simulink model "CORDIC"  (R2021a)
settings: Solver=VariableStepAuto  StartTime=0.0  StopTime=400  RelTol=1e-3
undefined symbols (not defined in the file or in its folder): AXI4, Lite
libraries: hdlBasic x776, xbsIndex_r4 x1
(part 7 of 7)

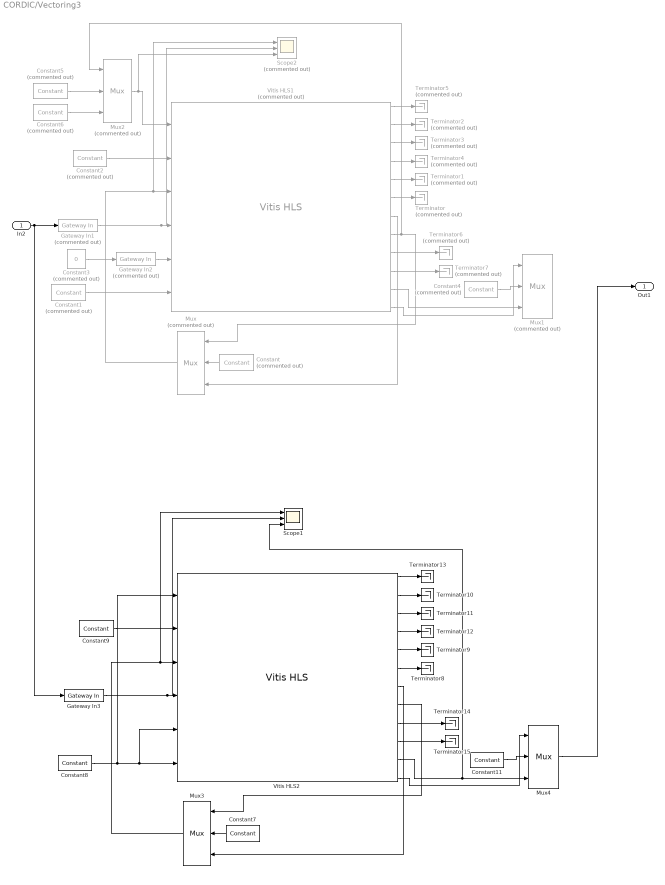
== system CORDIC/Vectoring3 ==
  In2 : Inport
  Constant : hdlBasic/Constant  Commented=on  const=0  gui_display_data_type=Fixed-point  arith_type=Signed (2's comp)  n_bits=16  bin_pt=13  preci_type=Single  exp_width=8  frac_width=24  explicit_period=off  period=1  XmcBlockStatus=1  maskContainerNames=tabcontainer1  block_type=constant  block_config=sysgen:Constant_config
  Constant1 : hdlBasic/Constant  Commented=on  const=0  gui_display_data_type=Boolean  arith_type=Boolean  n_bits=16  bin_pt=13  preci_type=Single  exp_width=8  frac_width=24  explicit_period=off  period=1  XmcBlockStatus=1  maskContainerNames=tabcontainer1  block_type=constant  block_config=sysgen:Constant_config
  Constant11 : hdlBasic/Constant  const=0  gui_display_data_type=Fixed-point  arith_type=Signed (2's comp)  n_bits=16  bin_pt=13  preci_type=Single  exp_width=8  frac_width=24  explicit_period=off  period=1  XmcBlockStatus=1  maskContainerNames=tabcontainer1  block_type=constant  block_config=sysgen:Constant_config
  Constant2 : hdlBasic/Constant  Commented=on  const=1  gui_display_data_type=Boolean  arith_type=Boolean  n_bits=16  bin_pt=13  preci_type=Single  exp_width=8  frac_width=24  explicit_period=off  period=1  XmcBlockStatus=1  maskContainerNames=tabcontainer1  block_type=constant  block_config=sysgen:Constant_config
  Constant3 : Constant  Commented=on  Value=0
  Constant4 : hdlBasic/Constant  Commented=on  const=0  gui_display_data_type=Fixed-point  arith_type=Signed (2's comp)  n_bits=16  bin_pt=13  preci_type=Single  exp_width=8  frac_width=24  explicit_period=off  period=1  XmcBlockStatus=1  maskContainerNames=tabcontainer1  block_type=constant  block_config=sysgen:Constant_config
  Constant5 : hdlBasic/Constant  Commented=on  const=0  gui_display_data_type=Boolean  arith_type=Boolean  n_bits=16  bin_pt=14  preci_type=Single  exp_width=8  frac_width=24  explicit_period=off  period=1  XmcBlockStatus=1  maskContainerNames=tabcontainer1  block_type=constant  block_config=sysgen:Constant_config
  Constant6 : hdlBasic/Constant  Commented=on  const=1.0  gui_display_data_type=Boolean  arith_type=Boolean  n_bits=16  bin_pt=14  preci_type=Single  exp_width=8  frac_width=24  explicit_period=off  period=1  XmcBlockStatus=1  maskContainerNames=tabcontainer1  block_type=constant  block_config=sysgen:Constant_config
  Constant7 : hdlBasic/Constant  const=0  gui_display_data_type=Fixed-point  arith_type=Signed (2's comp)  n_bits=16  bin_pt=13  preci_type=Single  exp_width=8  frac_width=24  explicit_period=off  period=1  XmcBlockStatus=1  maskContainerNames=tabcontainer1  block_type=constant  block_config=sysgen:Constant_config
  Constant8 : hdlBasic/Constant  const=0  gui_display_data_type=Boolean  arith_type=Boolean  n_bits=16  bin_pt=13  preci_type=Single  exp_width=8  frac_width=24  explicit_period=off  period=1  XmcBlockStatus=1  maskContainerNames=tabcontainer1  block_type=constant  block_config=sysgen:Constant_config
  Constant9 : hdlBasic/Constant  const=1  gui_display_data_type=Boolean  arith_type=Boolean  n_bits=16  bin_pt=13  preci_type=Single  exp_width=8  frac_width=24  explicit_period=off  period=1  XmcBlockStatus=1  maskContainerNames=tabcontainer1  block_type=constant  block_config=sysgen:Constant_config
  Gateway In1 : hdlBasic/Gateway In  Commented=on  gui_display_data_type=Fixed-point  arith_type=Signed (2's comp)  n_bits=16  bin_pt=13  preci_type=Single  exp_width=8  frac_width=24  rows=1  columns=1  quantization="Round  (unbiased: +/- Inf)"  overflow=Saturate  period=1  UseAsADC=off  ADCChannel='1'  interface=None  automatic_assignment=on  address_offset=hex2dec('00')  intf_name=''  intf_description=''  default_value=0  timing_constraint=None  locs_specified=off  LOCs={}  io_standard={}  inherit_from_input=off  hdl_port=on  XmcBlockStatus=1  maskContainerNames=group4  block_type=gatewayin  block_config=sysgen:gateway_in_config  block_width_w=590  block_height_w=620  block_width=640  block_height=850
  Gateway In2 : hdlBasic/Gateway In  Commented=on  gui_display_data_type=Fixed-point  arith_type=Signed (2's comp)  n_bits=16  bin_pt=13  preci_type=Single  exp_width=8  frac_width=24  rows=1  columns=1  quantization="Round  (unbiased: +/- Inf)"  overflow=Saturate  period=1  UseAsADC=off  ADCChannel='1'  interface=None  automatic_assignment=on  address_offset=hex2dec('00')  intf_name=''  intf_description=''  default_value=0  timing_constraint=None  locs_specified=off  LOCs={}  io_standard={}  inherit_from_input=off  hdl_port=on  XmcBlockStatus=1  maskContainerNames=group4  block_type=gatewayin  block_config=sysgen:gateway_in_config  block_width_w=590  block_height_w=620  block_width=640  block_height=850
  Gateway In3 : hdlBasic/Gateway In  gui_display_data_type=Fixed-point  arith_type=Signed (2's comp)  n_bits=16  bin_pt=13  preci_type=Single  exp_width=8  frac_width=24  rows=1  columns=1  quantization="Round  (unbiased: +/- Inf)"  overflow=Saturate  period=1  UseAsADC=off  ADCChannel='1'  interface=None  automatic_assignment=on  address_offset=hex2dec('00')  intf_name=''  intf_description=''  default_value=0  timing_constraint=None  locs_specified=off  LOCs={}  io_standard={}  inherit_from_input=off  hdl_port=on  XmcBlockStatus=1  maskContainerNames=group4  block_type=gatewayin  block_config=sysgen:gateway_in_config  block_width_w=590  block_height_w=620  block_width=640  block_height=850
  Mux : hdlBasic/Mux  Commented=on  inputs=2  en=off  latency=1  precision=Full  arith_type=Unsigned  n_bits=16  bin_pt=14  quantization=Truncate  overflow=Wrap  XmcBlockStatus=1  maskContainerNames=tabcontainer1  block_type=mux  block_config=sysgen:Mux_config
  Mux1 : hdlBasic/Mux  Commented=on  inputs=2  en=off  latency=1  precision=Full  arith_type=Unsigned  n_bits=16  bin_pt=14  quantization=Truncate  overflow=Wrap  XmcBlockStatus=1  maskContainerNames=tabcontainer1  block_type=mux  block_config=sysgen:Mux_config
  Mux2 : hdlBasic/Mux  Commented=on  inputs=2  en=off  latency=1  precision=Full  arith_type=Unsigned  n_bits=16  bin_pt=14  quantization=Truncate  overflow=Wrap  XmcBlockStatus=1  maskContainerNames=tabcontainer1  block_type=mux  block_config=sysgen:Mux_config
  Mux3 : hdlBasic/Mux  inputs=2  en=off  latency=1  precision=Full  arith_type=Unsigned  n_bits=16  bin_pt=14  quantization=Truncate  overflow=Wrap  XmcBlockStatus=1  maskContainerNames=tabcontainer1  block_type=mux  block_config=sysgen:Mux_config
  Mux4 : hdlBasic/Mux  inputs=2  en=off  latency=1  precision=Full  arith_type=Unsigned  n_bits=16  bin_pt=14  quantization=Truncate  overflow=Wrap  XmcBlockStatus=1  maskContainerNames=tabcontainer1  block_type=mux  block_config=sysgen:Mux_config
  Scope1 : Scope  NumInputPorts=3
  Scope2 : Scope  Commented=on  NumInputPorts=3
  Terminator{,1..7} (8 alike) : Terminator  Commented=on
  Terminator{8..15} (8 alike) : Terminator
  Vitis HLS1 : hdlBasic/Vitis HLS  Commented=on  anytable='C:\ELEC522\jz118\HLS\cordic\solution1'  fast_sim=off  display_datatype=off  rate_propagation_method=Simulink system period  model_file_path=''  latency=1  block_type=vitis_hls
      settings: infoedit=This block allows including C,C++ and SystemC source files in System Generator for DSP designs.
  Vitis HLS2 : hdlBasic/Vitis HLS  anytable='C:\ELEC522\jz118\HLS\cordic\solution1'  fast_sim=off  display_datatype=off  rate_propagation_method=Simulink system period  model_file_path=''  latency=1  block_type=vitis_hls
      settings: infoedit=This block allows including C,C++ and SystemC source files in System Generator for DSP designs.
  Out1 : Outport
  wires:
  Gateway In2/1 -> Vitis HLS1/5
  In2/1 -> Gateway In1/1, Gateway In3/1
  Gateway In1/1 -> Scope2/2, Vitis HLS1/4
  Constant3/1 -> Gateway In2/1
  Constant2/1 -> Vitis HLS1/2
  Vitis HLS1/8 -> Mux/1, Mux2/1
  Mux/1 -> Scope2/1, Vitis HLS1/3
  Constant/1 -> Mux/2
  Vitis HLS1/7 -> Mux/3
  Vitis HLS1/6 -> Terminator/1
  Vitis HLS1/5 -> Terminator1/1
  Vitis HLS1/2 -> Terminator2/1
  Vitis HLS1/3 -> Terminator3/1
  Vitis HLS1/4 -> Terminator4/1
  Vitis HLS1/1 -> Terminator5/1
  Vitis HLS1/9 -> Terminator6/1
  Vitis HLS1/10 -> Terminator7/1
  Vitis HLS1/11 -> Mux1/3
  Constant4/1 -> Mux1/2
  Vitis HLS1/12 -> Mux1/1
  Constant6/1 -> Mux2/3
  Constant5/1 -> Mux2/2
  Constant1/1 -> Vitis HLS1/6
  Mux2/1 -> Scope2/3, Vitis HLS1/1
  Constant11/1 -> Mux4/2
  Vitis HLS2/11 -> Scope1/3, Mux4/3
  Vitis HLS2/12 -> Mux4/1
  Vitis HLS2/9 -> Terminator14/1
  Vitis HLS2/5 -> Terminator9/1
  Vitis HLS2/2 -> Terminator10/1
  Vitis HLS2/4 -> Terminator12/1
  Vitis HLS2/6 -> Terminator8/1
  Vitis HLS2/10 -> Terminator15/1
  Constant7/1 -> Mux3/2
  Constant8/1 -> Vitis HLS2/1, Vitis HLS2/5, Vitis HLS2/6
  Mux3/1 -> Scope1/1, Vitis HLS2/3
  Vitis HLS2/7 -> Mux3/3
  Vitis HLS2/8 -> Mux3/1
  Gateway In3/1 -> Scope1/2, Vitis HLS2/4
  Constant9/1 -> Vitis HLS2/2
  Vitis HLS2/3 -> Terminator11/1
  Vitis HLS2/1 -> Terminator13/1
  Mux4/1 -> Out1/1

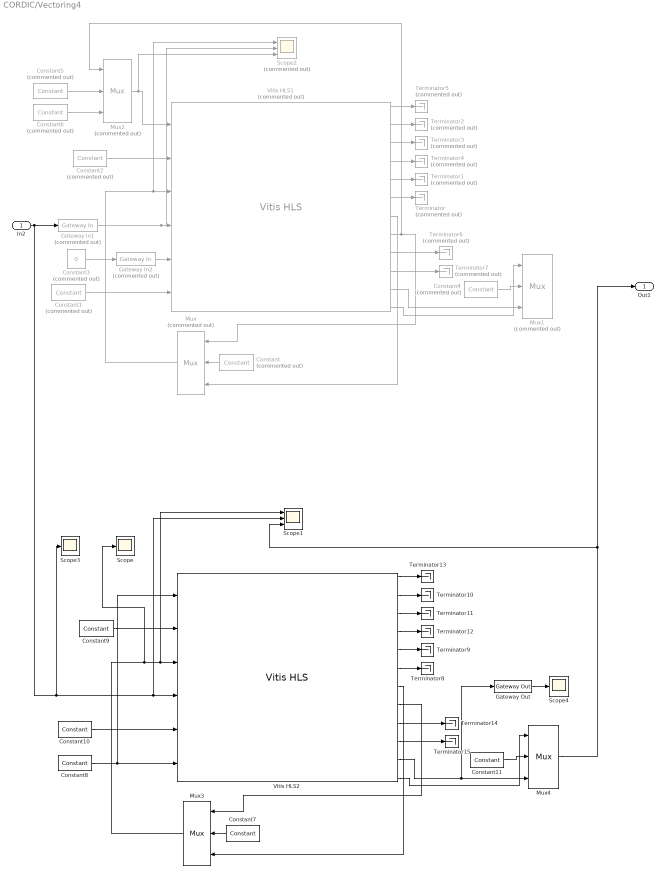
== system CORDIC/Vectoring4 ==
  In2 : Inport
  Constant : hdlBasic/Constant  Commented=on  const=0  gui_display_data_type=Fixed-point  arith_type=Signed (2's comp)  n_bits=16  bin_pt=13  preci_type=Single  exp_width=8  frac_width=24  explicit_period=off  period=1  XmcBlockStatus=1  maskContainerNames=tabcontainer1  block_type=constant  block_config=sysgen:Constant_config
  Constant1 : hdlBasic/Constant  Commented=on  const=0  gui_display_data_type=Boolean  arith_type=Boolean  n_bits=16  bin_pt=13  preci_type=Single  exp_width=8  frac_width=24  explicit_period=off  period=1  XmcBlockStatus=1  maskContainerNames=tabcontainer1  block_type=constant  block_config=sysgen:Constant_config
  Constant10 : hdlBasic/Constant  const=0  gui_display_data_type=Fixed-point  arith_type=Signed (2's comp)  n_bits=16  bin_pt=13  preci_type=Single  exp_width=8  frac_width=24  explicit_period=off  period=1  XmcBlockStatus=1  maskContainerNames=tabcontainer1  block_type=constant  block_config=sysgen:Constant_config
  Constant11 : hdlBasic/Constant  const=0  gui_display_data_type=Fixed-point  arith_type=Signed (2's comp)  n_bits=16  bin_pt=13  preci_type=Single  exp_width=8  frac_width=24  explicit_period=off  period=1  XmcBlockStatus=1  maskContainerNames=tabcontainer1  block_type=constant  block_config=sysgen:Constant_config
  Constant2 : hdlBasic/Constant  Commented=on  const=1  gui_display_data_type=Boolean  arith_type=Boolean  n_bits=16  bin_pt=13  preci_type=Single  exp_width=8  frac_width=24  explicit_period=off  period=1  XmcBlockStatus=1  maskContainerNames=tabcontainer1  block_type=constant  block_config=sysgen:Constant_config
  Constant3 : Constant  Commented=on  Value=0
  Constant4 : hdlBasic/Constant  Commented=on  const=0  gui_display_data_type=Fixed-point  arith_type=Signed (2's comp)  n_bits=16  bin_pt=13  preci_type=Single  exp_width=8  frac_width=24  explicit_period=off  period=1  XmcBlockStatus=1  maskContainerNames=tabcontainer1  block_type=constant  block_config=sysgen:Constant_config
  Constant5 : hdlBasic/Constant  Commented=on  const=0  gui_display_data_type=Boolean  arith_type=Boolean  n_bits=16  bin_pt=14  preci_type=Single  exp_width=8  frac_width=24  explicit_period=off  period=1  XmcBlockStatus=1  maskContainerNames=tabcontainer1  block_type=constant  block_config=sysgen:Constant_config
  Constant6 : hdlBasic/Constant  Commented=on  const=1.0  gui_display_data_type=Boolean  arith_type=Boolean  n_bits=16  bin_pt=14  preci_type=Single  exp_width=8  frac_width=24  explicit_period=off  period=1  XmcBlockStatus=1  maskContainerNames=tabcontainer1  block_type=constant  block_config=sysgen:Constant_config
  Constant7 : hdlBasic/Constant  const=0  gui_display_data_type=Fixed-point  arith_type=Signed (2's comp)  n_bits=16  bin_pt=13  preci_type=Single  exp_width=8  frac_width=24  explicit_period=off  period=1  XmcBlockStatus=1  maskContainerNames=tabcontainer1  block_type=constant  block_config=sysgen:Constant_config
  Constant8 : hdlBasic/Constant  const=0  gui_display_data_type=Boolean  arith_type=Boolean  n_bits=16  bin_pt=13  preci_type=Single  exp_width=8  frac_width=24  explicit_period=off  period=1  XmcBlockStatus=1  maskContainerNames=tabcontainer1  block_type=constant  block_config=sysgen:Constant_config
  Constant9 : hdlBasic/Constant  const=1  gui_display_data_type=Boolean  arith_type=Boolean  n_bits=16  bin_pt=13  preci_type=Single  exp_width=8  frac_width=24  explicit_period=off  period=1  XmcBlockStatus=1  maskContainerNames=tabcontainer1  block_type=constant  block_config=sysgen:Constant_config
  Gateway In1 : hdlBasic/Gateway In  Commented=on  gui_display_data_type=Fixed-point  arith_type=Signed (2's comp)  n_bits=16  bin_pt=13  preci_type=Single  exp_width=8  frac_width=24  rows=1  columns=1  quantization="Round  (unbiased: +/- Inf)"  overflow=Saturate  period=1  UseAsADC=off  ADCChannel='1'  interface=None  automatic_assignment=on  address_offset=hex2dec('00')  intf_name=''  intf_description=''  default_value=0  timing_constraint=None  locs_specified=off  LOCs={}  io_standard={}  inherit_from_input=off  hdl_port=on  XmcBlockStatus=1  maskContainerNames=group4  block_type=gatewayin  block_config=sysgen:gateway_in_config  block_width_w=590  block_height_w=620  block_width=640  block_height=850
  Gateway In2 : hdlBasic/Gateway In  Commented=on  gui_display_data_type=Fixed-point  arith_type=Signed (2's comp)  n_bits=16  bin_pt=13  preci_type=Single  exp_width=8  frac_width=24  rows=1  columns=1  quantization="Round  (unbiased: +/- Inf)"  overflow=Saturate  period=1  UseAsADC=off  ADCChannel='1'  interface=None  automatic_assignment=on  address_offset=hex2dec('00')  intf_name=''  intf_description=''  default_value=0  timing_constraint=None  locs_specified=off  LOCs={}  io_standard={}  inherit_from_input=off  hdl_port=on  XmcBlockStatus=1  maskContainerNames=group4  block_type=gatewayin  block_config=sysgen:gateway_in_config  block_width_w=590  block_height_w=620  block_width=640  block_height=850
  Gateway Out : hdlBasic/Gateway Out  inherit_from_input=off  hdl_port=on  rows=1  columns=1  UseAsDAC=off  DACChannel='1'  interface=None  automatic_assignment=on  address_offset=hex2dec('00')  intf_name=''  intf_description=''  timing_constraint=None  locs_specified=off  LOCs={}  io_standard={}  XmcBlockStatus=1  maskContainerNames=group4  block_type=gatewayout  block_config=sysgen:gateway_out_config  block_width_w=590  block_height_w=620  block_width=620  block_height=750
  Mux : hdlBasic/Mux  Commented=on  inputs=2  en=off  latency=1  precision=Full  arith_type=Unsigned  n_bits=16  bin_pt=14  quantization=Truncate  overflow=Wrap  XmcBlockStatus=1  maskContainerNames=tabcontainer1  block_type=mux  block_config=sysgen:Mux_config
  Mux1 : hdlBasic/Mux  Commented=on  inputs=2  en=off  latency=1  precision=Full  arith_type=Unsigned  n_bits=16  bin_pt=14  quantization=Truncate  overflow=Wrap  XmcBlockStatus=1  maskContainerNames=tabcontainer1  block_type=mux  block_config=sysgen:Mux_config
  Mux2 : hdlBasic/Mux  Commented=on  inputs=2  en=off  latency=1  precision=Full  arith_type=Unsigned  n_bits=16  bin_pt=14  quantization=Truncate  overflow=Wrap  XmcBlockStatus=1  maskContainerNames=tabcontainer1  block_type=mux  block_config=sysgen:Mux_config
  Mux3 : hdlBasic/Mux  inputs=2  en=off  latency=1  precision=Full  arith_type=Unsigned  n_bits=16  bin_pt=14  quantization=Truncate  overflow=Wrap  XmcBlockStatus=1  maskContainerNames=tabcontainer1  block_type=mux  block_config=sysgen:Mux_config
  Mux4 : hdlBasic/Mux  inputs=2  en=off  latency=1  precision=Full  arith_type=Unsigned  n_bits=16  bin_pt=14  quantization=Truncate  overflow=Wrap  XmcBlockStatus=1  maskContainerNames=tabcontainer1  block_type=mux  block_config=sysgen:Mux_config
  Scope : Scope
  Scope1 : Scope  NumInputPorts=3
  Scope2 : Scope  Commented=on  NumInputPorts=3
  Scope3 : Scope
  Scope4 : Scope
  Terminator{,1..7} (8 alike) : Terminator  Commented=on
  Terminator{8..15} (8 alike) : Terminator
  Vitis HLS1 : hdlBasic/Vitis HLS  Commented=on  anytable='C:\ELEC522\jz118\HLS\cordic\solution1'  fast_sim=off  display_datatype=off  rate_propagation_method=Simulink system period  model_file_path=''  latency=1  block_type=vitis_hls
      settings: infoedit=This block allows including C,C++ and SystemC source files in System Generator for DSP designs.
  Vitis HLS2 : hdlBasic/Vitis HLS  anytable='C:\ELEC522\jz118\HLS\cordic\solution1'  fast_sim=off  display_datatype=off  rate_propagation_method=Simulink system period  model_file_path=''  latency=1  block_type=vitis_hls
      settings: infoedit=This block allows including C,C++ and SystemC source files in System Generator for DSP designs.
  Out1 : Outport
  wires:
  Gateway In2/1 -> Vitis HLS1/5
  Gateway In1/1 -> Scope2/2, Vitis HLS1/4
  Constant3/1 -> Gateway In2/1
  Constant2/1 -> Vitis HLS1/2
  Vitis HLS1/8 -> Mux/1, Mux2/1
  Mux/1 -> Scope2/1, Vitis HLS1/3
  Constant/1 -> Mux/2
  Vitis HLS1/7 -> Mux/3
  Vitis HLS1/6 -> Terminator/1
  Vitis HLS1/5 -> Terminator1/1
  Vitis HLS1/2 -> Terminator2/1
  Vitis HLS1/3 -> Terminator3/1
  Vitis HLS1/4 -> Terminator4/1
  Vitis HLS1/1 -> Terminator5/1
  Vitis HLS1/9 -> Terminator6/1
  Vitis HLS1/10 -> Terminator7/1
  Vitis HLS1/11 -> Mux1/3
  Constant4/1 -> Mux1/2
  Vitis HLS1/12 -> Mux1/1
  Constant6/1 -> Mux2/3
  Constant5/1 -> Mux2/2
  Constant1/1 -> Vitis HLS1/6
  Mux2/1 -> Scope2/3, Vitis HLS1/1
  Constant11/1 -> Mux4/2
  Vitis HLS2/11 -> Gateway Out/1, Mux4/3
  Vitis HLS2/12 -> Mux4/1
  Vitis HLS2/9 -> Terminator14/1
  Vitis HLS2/5 -> Terminator9/1
  Vitis HLS2/2 -> Terminator10/1
  Vitis HLS2/4 -> Terminator12/1
  Vitis HLS2/6 -> Terminator8/1
  Vitis HLS2/10 -> Terminator15/1
  Constant7/1 -> Mux3/2
  Constant8/1 -> Vitis HLS2/1, Vitis HLS2/6
  Mux3/1 -> Scope/1, Scope1/1, Vitis HLS2/3
  Vitis HLS2/7 -> Mux3/3
  Vitis HLS2/8 -> Mux3/1
  Constant9/1 -> Vitis HLS2/2
  Vitis HLS2/3 -> Terminator11/1
  Vitis HLS2/1 -> Terminator13/1
  Mux4/1 -> Scope1/3, Out1/1
  Constant10/1 -> Vitis HLS2/5
  Gateway Out/1 -> Scope4/1
  In2/1 -> Scope1/2, Vitis HLS2/4, Scope3/1, Gateway In1/1

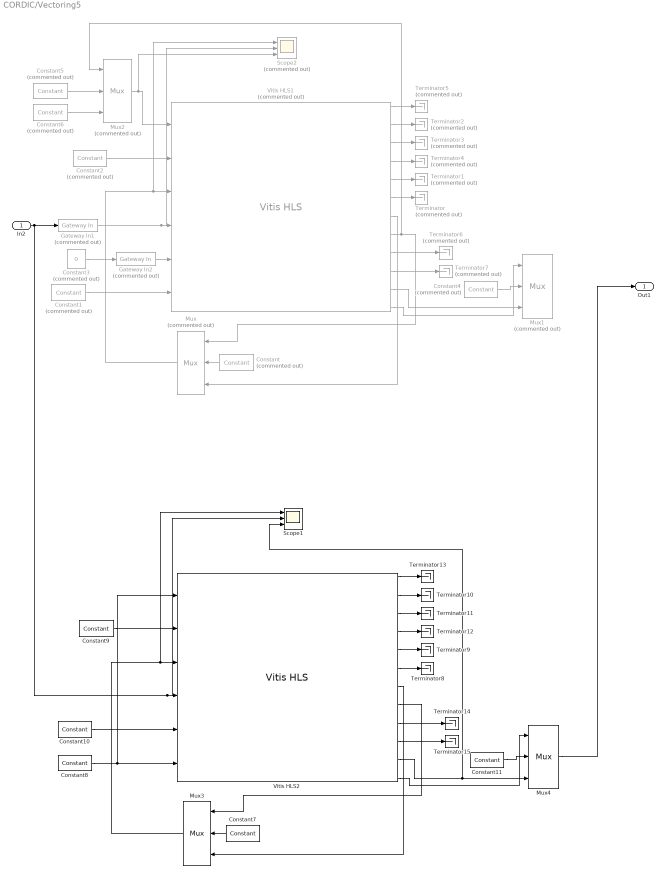
== system CORDIC/Vectoring5 ==
  In2 : Inport
  Constant : hdlBasic/Constant  Commented=on  const=0  gui_display_data_type=Fixed-point  arith_type=Signed (2's comp)  n_bits=16  bin_pt=13  preci_type=Single  exp_width=8  frac_width=24  explicit_period=off  period=1  XmcBlockStatus=1  maskContainerNames=tabcontainer1  block_type=constant  block_config=sysgen:Constant_config
  Constant1 : hdlBasic/Constant  Commented=on  const=0  gui_display_data_type=Boolean  arith_type=Boolean  n_bits=16  bin_pt=13  preci_type=Single  exp_width=8  frac_width=24  explicit_period=off  period=1  XmcBlockStatus=1  maskContainerNames=tabcontainer1  block_type=constant  block_config=sysgen:Constant_config
  Constant10 : hdlBasic/Constant  const=0  gui_display_data_type=Fixed-point  arith_type=Signed (2's comp)  n_bits=16  bin_pt=13  preci_type=Single  exp_width=8  frac_width=24  explicit_period=off  period=1  XmcBlockStatus=1  maskContainerNames=tabcontainer1  block_type=constant  block_config=sysgen:Constant_config
  Constant11 : hdlBasic/Constant  const=0  gui_display_data_type=Fixed-point  arith_type=Signed (2's comp)  n_bits=16  bin_pt=13  preci_type=Single  exp_width=8  frac_width=24  explicit_period=off  period=1  XmcBlockStatus=1  maskContainerNames=tabcontainer1  block_type=constant  block_config=sysgen:Constant_config
  Constant2 : hdlBasic/Constant  Commented=on  const=1  gui_display_data_type=Boolean  arith_type=Boolean  n_bits=16  bin_pt=13  preci_type=Single  exp_width=8  frac_width=24  explicit_period=off  period=1  XmcBlockStatus=1  maskContainerNames=tabcontainer1  block_type=constant  block_config=sysgen:Constant_config
  Constant3 : Constant  Commented=on  Value=0
  Constant4 : hdlBasic/Constant  Commented=on  const=0  gui_display_data_type=Fixed-point  arith_type=Signed (2's comp)  n_bits=16  bin_pt=13  preci_type=Single  exp_width=8  frac_width=24  explicit_period=off  period=1  XmcBlockStatus=1  maskContainerNames=tabcontainer1  block_type=constant  block_config=sysgen:Constant_config
  Constant5 : hdlBasic/Constant  Commented=on  const=0  gui_display_data_type=Boolean  arith_type=Boolean  n_bits=16  bin_pt=14  preci_type=Single  exp_width=8  frac_width=24  explicit_period=off  period=1  XmcBlockStatus=1  maskContainerNames=tabcontainer1  block_type=constant  block_config=sysgen:Constant_config
  Constant6 : hdlBasic/Constant  Commented=on  const=1.0  gui_display_data_type=Boolean  arith_type=Boolean  n_bits=16  bin_pt=14  preci_type=Single  exp_width=8  frac_width=24  explicit_period=off  period=1  XmcBlockStatus=1  maskContainerNames=tabcontainer1  block_type=constant  block_config=sysgen:Constant_config
  Constant7 : hdlBasic/Constant  const=0  gui_display_data_type=Fixed-point  arith_type=Signed (2's comp)  n_bits=16  bin_pt=13  preci_type=Single  exp_width=8  frac_width=24  explicit_period=off  period=1  XmcBlockStatus=1  maskContainerNames=tabcontainer1  block_type=constant  block_config=sysgen:Constant_config
  Constant8 : hdlBasic/Constant  const=0  gui_display_data_type=Boolean  arith_type=Boolean  n_bits=16  bin_pt=13  preci_type=Single  exp_width=8  frac_width=24  explicit_period=off  period=1  XmcBlockStatus=1  maskContainerNames=tabcontainer1  block_type=constant  block_config=sysgen:Constant_config
  Constant9 : hdlBasic/Constant  const=1  gui_display_data_type=Boolean  arith_type=Boolean  n_bits=16  bin_pt=13  preci_type=Single  exp_width=8  frac_width=24  explicit_period=off  period=1  XmcBlockStatus=1  maskContainerNames=tabcontainer1  block_type=constant  block_config=sysgen:Constant_config
  Gateway In1 : hdlBasic/Gateway In  Commented=on  gui_display_data_type=Fixed-point  arith_type=Signed (2's comp)  n_bits=16  bin_pt=13  preci_type=Single  exp_width=8  frac_width=24  rows=1  columns=1  quantization="Round  (unbiased: +/- Inf)"  overflow=Saturate  period=1  UseAsADC=off  ADCChannel='1'  interface=None  automatic_assignment=on  address_offset=hex2dec('00')  intf_name=''  intf_description=''  default_value=0  timing_constraint=None  locs_specified=off  LOCs={}  io_standard={}  inherit_from_input=off  hdl_port=on  XmcBlockStatus=1  maskContainerNames=group4  block_type=gatewayin  block_config=sysgen:gateway_in_config  block_width_w=590  block_height_w=620  block_width=640  block_height=850
  Gateway In2 : hdlBasic/Gateway In  Commented=on  gui_display_data_type=Fixed-point  arith_type=Signed (2's comp)  n_bits=16  bin_pt=13  preci_type=Single  exp_width=8  frac_width=24  rows=1  columns=1  quantization="Round  (unbiased: +/- Inf)"  overflow=Saturate  period=1  UseAsADC=off  ADCChannel='1'  interface=None  automatic_assignment=on  address_offset=hex2dec('00')  intf_name=''  intf_description=''  default_value=0  timing_constraint=None  locs_specified=off  LOCs={}  io_standard={}  inherit_from_input=off  hdl_port=on  XmcBlockStatus=1  maskContainerNames=group4  block_type=gatewayin  block_config=sysgen:gateway_in_config  block_width_w=590  block_height_w=620  block_width=640  block_height=850
  Mux : hdlBasic/Mux  Commented=on  inputs=2  en=off  latency=1  precision=Full  arith_type=Unsigned  n_bits=16  bin_pt=14  quantization=Truncate  overflow=Wrap  XmcBlockStatus=1  maskContainerNames=tabcontainer1  block_type=mux  block_config=sysgen:Mux_config
  Mux1 : hdlBasic/Mux  Commented=on  inputs=2  en=off  latency=1  precision=Full  arith_type=Unsigned  n_bits=16  bin_pt=14  quantization=Truncate  overflow=Wrap  XmcBlockStatus=1  maskContainerNames=tabcontainer1  block_type=mux  block_config=sysgen:Mux_config
  Mux2 : hdlBasic/Mux  Commented=on  inputs=2  en=off  latency=1  precision=Full  arith_type=Unsigned  n_bits=16  bin_pt=14  quantization=Truncate  overflow=Wrap  XmcBlockStatus=1  maskContainerNames=tabcontainer1  block_type=mux  block_config=sysgen:Mux_config
  Mux3 : hdlBasic/Mux  inputs=2  en=off  latency=1  precision=Full  arith_type=Unsigned  n_bits=16  bin_pt=14  quantization=Truncate  overflow=Wrap  XmcBlockStatus=1  maskContainerNames=tabcontainer1  block_type=mux  block_config=sysgen:Mux_config
  Mux4 : hdlBasic/Mux  inputs=2  en=off  latency=1  precision=Full  arith_type=Unsigned  n_bits=16  bin_pt=14  quantization=Truncate  overflow=Wrap  XmcBlockStatus=1  maskContainerNames=tabcontainer1  block_type=mux  block_config=sysgen:Mux_config
  Scope1 : Scope  NumInputPorts=3
  Scope2 : Scope  Commented=on  NumInputPorts=3
  Terminator{,1..7} (8 alike) : Terminator  Commented=on
  Terminator{8..15} (8 alike) : Terminator
  Vitis HLS1 : hdlBasic/Vitis HLS  Commented=on  anytable='C:\ELEC522\jz118\HLS\cordic\solution1'  fast_sim=off  display_datatype=off  rate_propagation_method=Simulink system period  model_file_path=''  latency=1  block_type=vitis_hls
      settings: infoedit=This block allows including C,C++ and SystemC source files in System Generator for DSP designs.
  Vitis HLS2 : hdlBasic/Vitis HLS  anytable='C:\ELEC522\jz118\HLS\cordic\solution1'  fast_sim=off  display_datatype=off  rate_propagation_method=Simulink system period  model_file_path=''  latency=1  block_type=vitis_hls
      settings: infoedit=This block allows including C,C++ and SystemC source files in System Generator for DSP designs.
  Out1 : Outport
  wires:
  Gateway In2/1 -> Vitis HLS1/5
  Gateway In1/1 -> Scope2/2, Vitis HLS1/4
  Constant3/1 -> Gateway In2/1
  Constant2/1 -> Vitis HLS1/2
  Vitis HLS1/8 -> Mux/1, Mux2/1
  Mux/1 -> Scope2/1, Vitis HLS1/3
  Constant/1 -> Mux/2
  Vitis HLS1/7 -> Mux/3
  Vitis HLS1/6 -> Terminator/1
  Vitis HLS1/5 -> Terminator1/1
  Vitis HLS1/2 -> Terminator2/1
  Vitis HLS1/3 -> Terminator3/1
  Vitis HLS1/4 -> Terminator4/1
  Vitis HLS1/1 -> Terminator5/1
  Vitis HLS1/9 -> Terminator6/1
  Vitis HLS1/10 -> Terminator7/1
  Vitis HLS1/11 -> Mux1/3
  Constant4/1 -> Mux1/2
  Vitis HLS1/12 -> Mux1/1
  Constant6/1 -> Mux2/3
  Constant5/1 -> Mux2/2
  Constant1/1 -> Vitis HLS1/6
  Mux2/1 -> Scope2/3, Vitis HLS1/1
  Constant11/1 -> Mux4/2
  Vitis HLS2/11 -> Scope1/3, Mux4/3
  Vitis HLS2/12 -> Mux4/1
  Vitis HLS2/9 -> Terminator14/1
  Vitis HLS2/5 -> Terminator9/1
  Vitis HLS2/2 -> Terminator10/1
  Vitis HLS2/4 -> Terminator12/1
  Vitis HLS2/6 -> Terminator8/1
  Vitis HLS2/10 -> Terminator15/1
  Constant7/1 -> Mux3/2
  Constant8/1 -> Vitis HLS2/1, Vitis HLS2/6
  Mux3/1 -> Scope1/1, Vitis HLS2/3
  Vitis HLS2/7 -> Mux3/3
  Vitis HLS2/8 -> Mux3/1
  In2/1 -> Scope1/2, Vitis HLS2/4, Gateway In1/1
  Constant9/1 -> Vitis HLS2/2
  Vitis HLS2/3 -> Terminator11/1
  Vitis HLS2/1 -> Terminator13/1
  Mux4/1 -> Out1/1
  Constant10/1 -> Vitis HLS2/5

== system CORDIC/Vectoring6 ==
  In2 : Inport
  Constant10 : hdlBasic/Constant  const=0  gui_display_data_type=Fixed-point  arith_type=Signed (2's comp)  n_bits=16  bin_pt=13  preci_type=Single  exp_width=8  frac_width=24  explicit_period=off  period=1  XmcBlockStatus=1  maskContainerNames=tabcontainer1  block_type=constant  block_config=sysgen:Constant_config
  Constant11 : hdlBasic/Constant  const=0  gui_display_data_type=Fixed-point  arith_type=Signed (2's comp)  n_bits=16  bin_pt=13  preci_type=Single  exp_width=8  frac_width=24  explicit_period=off  period=1  XmcBlockStatus=1  maskContainerNames=tabcontainer1  block_type=constant  block_config=sysgen:Constant_config
  Constant8 : hdlBasic/Constant  const=0  gui_display_data_type=Boolean  arith_type=Boolean  n_bits=16  bin_pt=13  preci_type=Single  exp_width=8  frac_width=24  explicit_period=off  period=1  XmcBlockStatus=1  maskContainerNames=tabcontainer1  block_type=constant  block_config=sysgen:Constant_config
  Constant9 : hdlBasic/Constant  const=1  gui_display_data_type=Boolean  arith_type=Boolean  n_bits=16  bin_pt=13  preci_type=Single  exp_width=8  frac_width=24  explicit_period=off  period=1  XmcBlockStatus=1  maskContainerNames=tabcontainer1  block_type=constant  block_config=sysgen:Constant_config
  Mux4 : hdlBasic/Mux  inputs=2  en=off  latency=1  precision=Full  arith_type=Unsigned  n_bits=16  bin_pt=14  quantization=Truncate  overflow=Wrap  XmcBlockStatus=1  maskContainerNames=tabcontainer1  block_type=mux  block_config=sysgen:Mux_config
  Register : hdlBasic/Register  init=0  rst=off  en=on  XmcBlockStatus=1  maskContainerNames=tabcontainer1  block_type=register  block_config=sysgen:Register_config
  Scope : Scope  NumInputPorts=2
  Terminator{8..15} (8 alike) : Terminator
  Vitis HLS2 : hdlBasic/Vitis HLS  anytable='C:\ELEC522\jz118\HLS\cordic\solution1'  fast_sim=off  display_datatype=off  rate_propagation_method=Simulink system period  model_file_path=''  latency=1  block_type=vitis_hls
      settings: infoedit=This block allows including C,C++ and SystemC source files in System Generator for DSP designs.
  Out1 : Outport
  Out2 : Outport  Port=2
  wires:
  Vitis HLS2/9 -> Terminator14/1
  Vitis HLS2/5 -> Terminator9/1
  Vitis HLS2/2 -> Terminator10/1
  Vitis HLS2/4 -> Terminator12/1
  Vitis HLS2/6 -> Terminator8/1
  Vitis HLS2/10 -> Terminator15/1
  Constant8/1 -> Vitis HLS2/1, Vitis HLS2/6
  Constant9/1 -> Vitis HLS2/2
  Vitis HLS2/3 -> Terminator11/1
  Vitis HLS2/1 -> Terminator13/1
  Constant10/1 -> Vitis HLS2/5
  In2/1 -> Scope/1, Vitis HLS2/4
  Vitis HLS2/7 -> Register/1
  Vitis HLS2/8 -> Register/2
  Register/1 -> Out2/1, Scope/2, Vitis HLS2/3
  Constant11/1 -> Mux4/2
  Mux4/1 -> Out1/1
  Vitis HLS2/12 -> Mux4/1
  Vitis HLS2/11 -> Mux4/3

== system CORDIC/Vectoring7 ==
  In2 : Inport
  Constant10 : hdlBasic/Constant  const=0  gui_display_data_type=Fixed-point  arith_type=Signed (2's comp)  n_bits=16  bin_pt=13  preci_type=Single  exp_width=8  frac_width=24  explicit_period=off  period=1  XmcBlockStatus=1  maskContainerNames=tabcontainer1  block_type=constant  block_config=sysgen:Constant_config
  Constant11 : hdlBasic/Constant  const=0  gui_display_data_type=Fixed-point  arith_type=Signed (2's comp)  n_bits=16  bin_pt=13  preci_type=Single  exp_width=8  frac_width=24  explicit_period=off  period=1  XmcBlockStatus=1  maskContainerNames=tabcontainer1  block_type=constant  block_config=sysgen:Constant_config
  Constant8 : hdlBasic/Constant  const=0  gui_display_data_type=Boolean  arith_type=Boolean  n_bits=16  bin_pt=13  preci_type=Single  exp_width=8  frac_width=24  explicit_period=off  period=1  XmcBlockStatus=1  maskContainerNames=tabcontainer1  block_type=constant  block_config=sysgen:Constant_config
  Constant9 : hdlBasic/Constant  const=1  gui_display_data_type=Boolean  arith_type=Boolean  n_bits=16  bin_pt=13  preci_type=Single  exp_width=8  frac_width=24  explicit_period=off  period=1  XmcBlockStatus=1  maskContainerNames=tabcontainer1  block_type=constant  block_config=sysgen:Constant_config
  Mux4 : hdlBasic/Mux  inputs=2  en=off  latency=1  precision=Full  arith_type=Unsigned  n_bits=16  bin_pt=14  quantization=Truncate  overflow=Wrap  XmcBlockStatus=1  maskContainerNames=tabcontainer1  block_type=mux  block_config=sysgen:Mux_config
  Register : hdlBasic/Register  init=0  rst=off  en=on  XmcBlockStatus=1  maskContainerNames=tabcontainer1  block_type=register  block_config=sysgen:Register_config
  Scope : Scope  NumInputPorts=2
  Terminator{8..15} (8 alike) : Terminator
  Vitis HLS2 : hdlBasic/Vitis HLS  anytable='C:\ELEC522\jz118\HLS\cordic\solution1'  fast_sim=off  display_datatype=off  rate_propagation_method=Simulink system period  model_file_path=''  latency=1  block_type=vitis_hls
      settings: infoedit=This block allows including C,C++ and SystemC source files in System Generator for DSP designs.
  Out1 : Outport
  Out2 : Outport  Port=2
  wires:
  Vitis HLS2/9 -> Terminator14/1
  Vitis HLS2/5 -> Terminator9/1
  Vitis HLS2/2 -> Terminator10/1
  Vitis HLS2/4 -> Terminator12/1
  Vitis HLS2/6 -> Terminator8/1
  Vitis HLS2/10 -> Terminator15/1
  Constant8/1 -> Vitis HLS2/1, Vitis HLS2/6
  Constant9/1 -> Vitis HLS2/2
  Vitis HLS2/3 -> Terminator11/1
  Vitis HLS2/1 -> Terminator13/1
  Constant10/1 -> Vitis HLS2/5
  In2/1 -> Scope/1, Vitis HLS2/4
  Vitis HLS2/7 -> Register/1
  Vitis HLS2/8 -> Register/2
  Register/1 -> Out2/1, Scope/2, Vitis HLS2/3
  Constant11/1 -> Mux4/2
  Vitis HLS2/11 -> Mux4/3
  Vitis HLS2/12 -> Mux4/1
  Mux4/1 -> Out1/1

== system CORDIC/Vectoring8 ==
  In1 : Inport
  In2 : Inport  Port=2
  Constant1 : hdlBasic/Constant  const=0  gui_display_data_type=Fixed-point  arith_type=Signed (2's comp)  n_bits=16  bin_pt=13  preci_type=Single  exp_width=8  frac_width=24  explicit_period=off  period=1  XmcBlockStatus=1  maskContainerNames=tabcontainer1  block_type=constant  block_config=sysgen:Constant_config
  Constant10 : hdlBasic/Constant  const=0  gui_display_data_type=Fixed-point  arith_type=Signed (2's comp)  n_bits=16  bin_pt=13  preci_type=Single  exp_width=8  frac_width=24  explicit_period=off  period=1  XmcBlockStatus=1  maskContainerNames=tabcontainer1  block_type=constant  block_config=sysgen:Constant_config
  Constant11 : hdlBasic/Constant  const=0  gui_display_data_type=Fixed-point  arith_type=Signed (2's comp)  n_bits=16  bin_pt=13  preci_type=Single  exp_width=8  frac_width=24  explicit_period=off  period=1  XmcBlockStatus=1  maskContainerNames=tabcontainer1  block_type=constant  block_config=sysgen:Constant_config
  Constant8 : hdlBasic/Constant  const=0  gui_display_data_type=Boolean  arith_type=Boolean  n_bits=16  bin_pt=13  preci_type=Single  exp_width=8  frac_width=24  explicit_period=off  period=1  XmcBlockStatus=1  maskContainerNames=tabcontainer1  block_type=constant  block_config=sysgen:Constant_config
  Constant9 : hdlBasic/Constant  const=1  gui_display_data_type=Boolean  arith_type=Boolean  n_bits=16  bin_pt=13  preci_type=Single  exp_width=8  frac_width=24  explicit_period=off  period=1  XmcBlockStatus=1  maskContainerNames=tabcontainer1  block_type=constant  block_config=sysgen:Constant_config
  Delay : hdlBasic/Delay  rst=off  en=off  latency=27  reg_retiming=off  XmcBlockStatus=1  maskContainerNames=group1  block_type=delay  block_config=sysgen:Delay_config
  Gateway Out43 : hdlBasic/Gateway Out  inherit_from_input=off  hdl_port=on  rows=1  columns=1  UseAsDAC=off  DACChannel='1'  interface=None  automatic_assignment=on  address_offset=hex2dec('00')  intf_name=''  intf_description=''  timing_constraint=None  locs_specified=off  LOCs={}  io_standard={}  XmcBlockStatus=1  maskContainerNames=group4  block_type=gatewayout  block_config=sysgen:gateway_out_config  block_width_w=590  block_height_w=620  block_width=620  block_height=750
  Mux : hdlBasic/Mux  inputs=2  en=off  latency=1  precision=Full  arith_type=Unsigned  n_bits=16  bin_pt=14  quantization=Truncate  overflow=Wrap  XmcBlockStatus=1  maskContainerNames=tabcontainer1  block_type=mux  block_config=sysgen:Mux_config
  Mux4 : hdlBasic/Mux  inputs=2  en=off  latency=1  precision=Full  arith_type=Unsigned  n_bits=16  bin_pt=14  quantization=Truncate  overflow=Wrap  XmcBlockStatus=1  maskContainerNames=tabcontainer1  block_type=mux  block_config=sysgen:Mux_config
  Register : hdlBasic/Register  init=0  rst=off  en=on  XmcBlockStatus=1  maskContainerNames=tabcontainer1  block_type=register  block_config=sysgen:Register_config
  Scope : Scope  NumInputPorts=2
  Terminator{8..15} (8 alike) : Terminator
  To Workspace12 : ToWorkspace  VariableName=simout12  SaveFormat=Timeseries  SampleTime=-1
  Vitis HLS2 : hdlBasic/Vitis HLS  anytable='C:\ELEC522\jz118\HLS\cordic\solution1'  fast_sim=off  display_datatype=off  rate_propagation_method=Simulink system period  model_file_path=''  latency=1  block_type=vitis_hls
      settings: infoedit=This block allows including C,C++ and SystemC source files in System Generator for DSP designs.
  Out1 : Outport
  Out3 : Outport  Port=2
  Out2 : Outport  Port=3
  wires:
  Vitis HLS2/9 -> Terminator14/1
  Vitis HLS2/5 -> Terminator9/1
  Vitis HLS2/2 -> Terminator10/1
  Vitis HLS2/4 -> Terminator12/1
  Vitis HLS2/6 -> Terminator8/1
  Vitis HLS2/10 -> Terminator15/1
  Constant8/1 -> Vitis HLS2/1, Vitis HLS2/6
  Constant9/1 -> Vitis HLS2/2
  Vitis HLS2/3 -> Terminator11/1
  Vitis HLS2/1 -> Terminator13/1
  Constant10/1 -> Vitis HLS2/5
  In2/1 -> Scope/1, Vitis HLS2/4
  Vitis HLS2/7 -> Register/1
  Vitis HLS2/8 -> Register/2
  Register/1 -> Mux/3, Scope/2, Vitis HLS2/3
  Constant11/1 -> Mux4/2
  Mux4/1 -> Out1/1
  Vitis HLS2/12 -> Mux4/1
  Vitis HLS2/11 -> Mux4/3
  In1/1 -> Delay/1, Mux/1
  Constant1/1 -> Mux/2
  Delay/1 -> Out3/1
  Gateway Out43/1 -> Out2/1, To Workspace12/1
  Mux/1 -> Gateway Out43/1

== system CORDIC/Vectoring9 ==
  In1 : Inport
  In2 : Inport  Port=2
  Constant1 : hdlBasic/Constant  const=0  gui_display_data_type=Fixed-point  arith_type=Signed (2's comp)  n_bits=16  bin_pt=13  preci_type=Single  exp_width=8  frac_width=24  explicit_period=off  period=1  XmcBlockStatus=1  maskContainerNames=tabcontainer1  block_type=constant  block_config=sysgen:Constant_config
  Constant10 : hdlBasic/Constant  const=0  gui_display_data_type=Fixed-point  arith_type=Signed (2's comp)  n_bits=16  bin_pt=13  preci_type=Single  exp_width=8  frac_width=24  explicit_period=off  period=1  XmcBlockStatus=1  maskContainerNames=tabcontainer1  block_type=constant  block_config=sysgen:Constant_config
  Constant11 : hdlBasic/Constant  const=0  gui_display_data_type=Fixed-point  arith_type=Signed (2's comp)  n_bits=16  bin_pt=13  preci_type=Single  exp_width=8  frac_width=24  explicit_period=off  period=1  XmcBlockStatus=1  maskContainerNames=tabcontainer1  block_type=constant  block_config=sysgen:Constant_config
  Constant8 : hdlBasic/Constant  const=0  gui_display_data_type=Boolean  arith_type=Boolean  n_bits=16  bin_pt=13  preci_type=Single  exp_width=8  frac_width=24  explicit_period=off  period=1  XmcBlockStatus=1  maskContainerNames=tabcontainer1  block_type=constant  block_config=sysgen:Constant_config
  Constant9 : hdlBasic/Constant  const=1  gui_display_data_type=Boolean  arith_type=Boolean  n_bits=16  bin_pt=13  preci_type=Single  exp_width=8  frac_width=24  explicit_period=off  period=1  XmcBlockStatus=1  maskContainerNames=tabcontainer1  block_type=constant  block_config=sysgen:Constant_config
  Delay : hdlBasic/Delay  rst=off  en=off  latency=27  reg_retiming=off  XmcBlockStatus=1  maskContainerNames=group1  block_type=delay  block_config=sysgen:Delay_config
  Gateway Out43 : hdlBasic/Gateway Out  inherit_from_input=off  hdl_port=on  rows=1  columns=1  UseAsDAC=off  DACChannel='1'  interface=None  automatic_assignment=on  address_offset=hex2dec('00')  intf_name=''  intf_description=''  timing_constraint=None  locs_specified=off  LOCs={}  io_standard={}  XmcBlockStatus=1  maskContainerNames=group4  block_type=gatewayout  block_config=sysgen:gateway_out_config  block_width_w=590  block_height_w=620  block_width=620  block_height=750
  Mux : hdlBasic/Mux  inputs=2  en=off  latency=1  precision=Full  arith_type=Unsigned  n_bits=16  bin_pt=14  quantization=Truncate  overflow=Wrap  XmcBlockStatus=1  maskContainerNames=tabcontainer1  block_type=mux  block_config=sysgen:Mux_config
  Mux4 : hdlBasic/Mux  inputs=2  en=off  latency=1  precision=Full  arith_type=Unsigned  n_bits=16  bin_pt=14  quantization=Truncate  overflow=Wrap  XmcBlockStatus=1  maskContainerNames=tabcontainer1  block_type=mux  block_config=sysgen:Mux_config
  Register : hdlBasic/Register  init=0  rst=off  en=on  XmcBlockStatus=1  maskContainerNames=tabcontainer1  block_type=register  block_config=sysgen:Register_config
  Scope : Scope  NumInputPorts=2
  Terminator{8..15} (8 alike) : Terminator
  To Workspace12 : ToWorkspace  VariableName=simout12  SaveFormat=Timeseries  SampleTime=-1
  Vitis HLS2 : hdlBasic/Vitis HLS  anytable='C:\ELEC522\jz118\HLS\cordic\solution1'  fast_sim=off  display_datatype=off  rate_propagation_method=Simulink system period  model_file_path=''  latency=1  block_type=vitis_hls
      settings: infoedit=This block allows including C,C++ and SystemC source files in System Generator for DSP designs.
  Out1 : Outport
  Out3 : Outport  Port=2
  Out2 : Outport  Port=3
  wires:
  Vitis HLS2/9 -> Terminator14/1
  Vitis HLS2/5 -> Terminator9/1
  Vitis HLS2/2 -> Terminator10/1
  Vitis HLS2/4 -> Terminator12/1
  Vitis HLS2/6 -> Terminator8/1
  Vitis HLS2/10 -> Terminator15/1
  Constant8/1 -> Vitis HLS2/1, Vitis HLS2/6
  Constant9/1 -> Vitis HLS2/2
  Vitis HLS2/3 -> Terminator11/1
  Vitis HLS2/1 -> Terminator13/1
  Constant10/1 -> Vitis HLS2/5
  In2/1 -> Scope/1, Vitis HLS2/4
  Vitis HLS2/7 -> Register/1
  Vitis HLS2/8 -> Register/2
  Register/1 -> Mux/3, Scope/2, Vitis HLS2/3
  Constant11/1 -> Mux4/2
  Mux4/1 -> Out1/1
  Vitis HLS2/12 -> Mux4/1
  Vitis HLS2/11 -> Mux4/3
  In1/1 -> Delay/1, Mux/1
  Constant1/1 -> Mux/2
  Delay/1 -> Out3/1
  Gateway Out43/1 -> Out2/1, To Workspace12/1
  Mux/1 -> Gateway Out43/1
